simulink model "ADCS_r2017b_may6"  (R2018a)
settings: Solver=VariableStepAuto  StartTime=0.0  StopTime=10.0  RelTol=1e-3
undefined symbols (not defined in the file or in its folder): delta_t, SC, SS
libraries: sharedutil x3, vrlib x2
(part 1 of 2)
settings Model: Creator=azufall  LastModifiedBy=Hridu

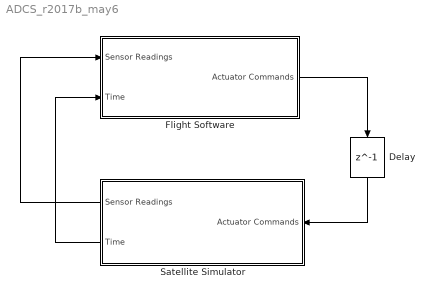
== system ADCS_r2017b_may6 ==
  Delay : Delay  DelayLength=1  InitialCondition=0
  Flight Software : Subsystem
  Satellite Simulator : Subsystem
  wires:
  Flight Software/1(Actuator Commands) -> Delay/1
  Satellite Simulator/2(Time) -> Flight Software/2(Time)
  Satellite Simulator/1(Sensor Readings) -> Flight Software/1(Sensor Readings)
  Delay/1 -> Satellite Simulator/1(Actuator Commands)

== system ADCS_r2017b_may6/Flight Software ==
  Sensor Readings : Inport
  Time : Inport  Port=2
  Bus Selector : BusSelector  OutputSignals=gyro meas,sun meas,star meas
  Resolution Error : Rounding
  Subsystems : Subsystem
  Thrust command : Gain
  Actuator Commands : Outport
  wires:
  Subsystems/1(RCS Command) -> Thrust command/1
  Sensor Readings/1 -> Bus Selector/1
  Bus Selector/1 -> Subsystems/1(Gyro)  "<gyro meas>"
  Bus Selector/3 -> Subsystems/3(Star Tracker)  "<star meas>"
  Time/1 -> Subsystems/4(Time)
  Thrust command/1 -> Resolution Error/1
  Resolution Error/1 -> Actuator Commands/1
  Bus Selector/2 -> Subsystems/2(Sun Sensor)  "<sun meas>"

== system ADCS_r2017b_may6/Satellite Simulator ==
  Actuator Commands : Inport
  Actuators : Subsystem
  Constant : Constant  Value=0
  Environment : Subsystem
  External Forces and Torques : Subsystem
  Kinematics : Subsystem
  Sensors : Subsystem
  Sum : Sum  Inputs=++|
  Sum1 : Sum  Inputs=++|
  Time Model : Subsystem
  Sensor Readings : Outport
  Time : Outport  Port=2
  wires:
  Kinematics/3(Omega) -> Sensors/3(w_body2eci)
  Sensors/1(Sensor Readings) -> Sensor Readings/1
  Time Model/1(JD) -> Kinematics/3(JD), Environment/1(Time), Time/1
  Environment/1(sun_eci) -> Sensors/2(Sun info), External Forces and Torques/4(sun_eci)
  Environment/2(moon_eci) -> External Forces and Torques/5(moon_eci)
  Environment/3(Mag) -> External Forces and Torques/6(Mag)
  External Forces and Torques/1(Ex Forces) -> Sum/2
  Sum/1 -> Kinematics/1(a_eci)
  External Forces and Torques/2(Ex Torques) -> Sum1/2
  Kinematics/2(Velocity) -> External Forces and Torques/2(Velocity)
  Kinematics/4(Coordinate Transforms) -> Environment/3(Coordinate Transforms), Sensors/4(Coordinate Transforms), Actuators/3(Coordinate Transforms), External Forces and Torques/3(Coordinate Transforms)
  Actuators/1(a_eci) -> Sum/1
  Actuators/2(torque_body) -> Sum1/1
  Sum1/1 -> Kinematics/2(Torque_body)
  Kinematics/1(Position) -> Sensors/1(Position), Environment/2(r_eci), External Forces and Torques/1(Position)
  Environment/4(Eclipse) -> Sensors/5(eclipse), External Forces and Torques/7(Eclipse)
  Kinematics/5(q) -> Sensors/6(q_eci2body)
  Actuator Commands/1 -> Actuators/1(RCS Command)
  Constant/1 -> Actuators/2(Other Actuator?)

== system ADCS_r2017b_may6/Flight Software/Subsystems ==
  Gyro : Inport
  Sun Sensor : Inport  Port=2
  Star Tracker : Inport  Port=3
  Time : Inport  Port=4
  Mode Selection : Subsystem
  RCS Controller : Subsystem
  Sensor Processing : Subsystem
  RCS Command : Outport
  wires:
  Gyro/1 -> Sensor Processing/1(Gyro_raw)
  Sun Sensor/1 -> Sensor Processing/2(Sun_raw)
  Star Tracker/1 -> Sensor Processing/3(Star_raw)
  Sensor Processing/1(Gyro_filtered) -> RCS Controller/2(Gyro), Mode Selection/1(Gyro)
  Sensor Processing/4(Eclipse) -> Mode Selection/2(Eclipse)
  Time/1 -> RCS Controller/6(Time), Mode Selection/3(Time)
  RCS Controller/1(RCS_Command) -> RCS Command/1
  Mode Selection/2(S/C Mode) -> RCS Controller/1(Mode)
  Mode Selection/1(Controller Gains) -> RCS Controller/5(Gains)
  Sensor Processing/3(Star_filtered) -> RCS Controller/4(Star)
  Sensor Processing/2(Sun_filtered) -> RCS Controller/3(Sun)

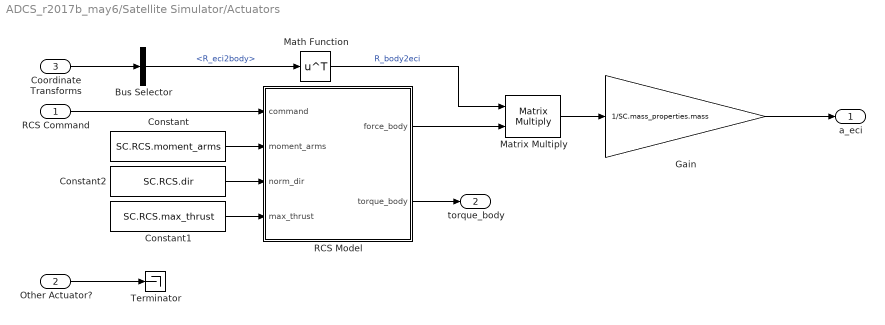
== system ADCS_r2017b_may6/Satellite Simulator/Actuators ==
  RCS Command : Inport
  Other Actuator? : Inport  Port=2
  Coordinate Transforms : Inport  Port=3
  Bus Selector : BusSelector  OutputSignals=R_eci2body
  Constant : Constant  Value=SC.RCS.moment_arms
  Constant1 : Constant  Value=SC.RCS.max_thrust
  Constant2 : Constant  Value=SC.RCS.dir
  Gain : Gain  Gain=1/SC.mass_properties.mass
  Math Function : Math  Operator=transpose  SaturateOnIntegerOverflow=on
  Matrix Multiply : Product  Multiplication=Matrix(*)
  RCS Model : MATLAB Function  TreatAsAtomicUnit=on
  Terminator : Terminator
  a_eci : Outport
  torque_body : Outport  Port=2
  wires:
  RCS Command/1 -> RCS Model/1(command)
  RCS Model/2(torque_body) -> torque_body/1
  Other Actuator?/1 -> Terminator/1
  Coordinate Transforms/1 -> Bus Selector/1
  Bus Selector/1 -> Math Function/1  "<R_eci2body>"
  RCS Model/1(force_body) -> Matrix Multiply/2
  Matrix Multiply/1 -> Gain/1
  Math Function/1 -> Matrix Multiply/1  "R_body2eci"
  Constant/1 -> RCS Model/2(moment_arms)
  Constant1/1 -> RCS Model/4(max_thrust)
  Constant2/1 -> RCS Model/3(norm_dir)
  Gain/1 -> a_eci/1

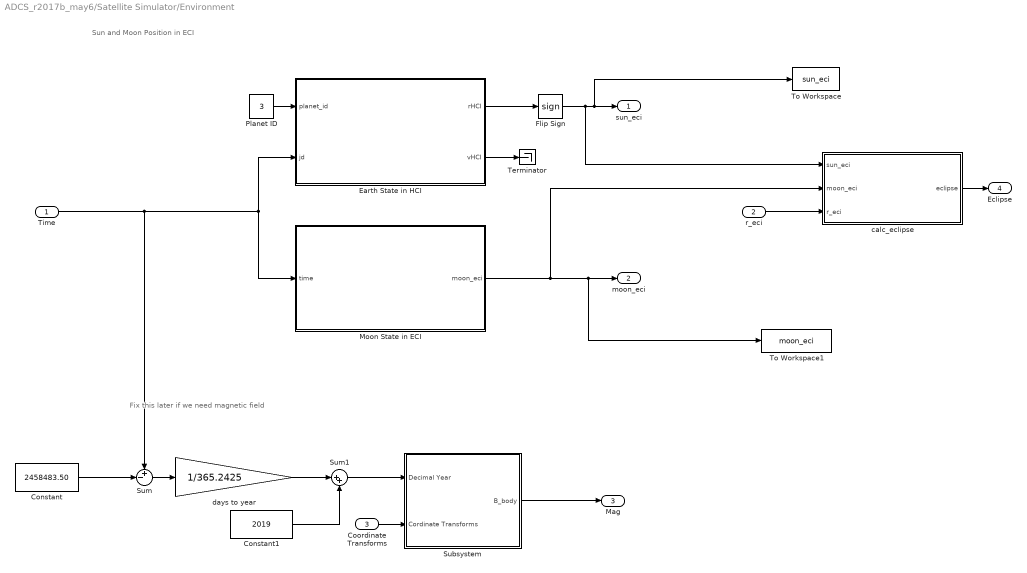
== system ADCS_r2017b_may6/Satellite Simulator/Environment ==
  note: Sun and Moon Position in ECI
  note: Fix this later if we need magnetic field
  Time : Inport
  r_eci : Inport  Port=2
  Coordinate Transforms : Inport  Port=3
  Constant : Constant  Value=2458483.50
  Constant1 : Constant  Value=2019
  Earth State in HCI : MATLAB Function  TreatAsAtomicUnit=on
  Flip Sign : Signum
  Moon State in ECI : MATLAB Function  TreatAsAtomicUnit=on
  Planet ID : Constant  Value=3
  Subsystem : Subsystem
  Sum : Sum  Inputs=+-|
  Sum1 : Sum  Inputs=|++
  Terminator : Terminator
  To Workspace : ToWorkspace  VariableName=sun_eci  SampleTime=-1
  To Workspace1 : ToWorkspace  VariableName=moon_eci  SampleTime=-1
  calc_eclipse : MATLAB Function  TreatAsAtomicUnit=on
  days to year : Gain  Gain=1/365.2425
  sun_eci : Outport
  moon_eci : Outport  Port=2
  Mag : Outport  Port=3
  Eclipse : Outport  Port=4
  wires:
  Moon State in ECI/1(moon_eci) -> calc_eclipse/2(moon_eci), To Workspace1/1, moon_eci/1
  Subsystem/1(B_body) -> Mag/1
  calc_eclipse/1(eclipse) -> Eclipse/1
  Time/1 -> Sum/1, Earth State in HCI/2(jd), Moon State in ECI/1(time)
  Planet ID/1 -> Earth State in HCI/1(planet_id)
  Earth State in HCI/1(rHCI) -> Flip Sign/1
  Flip Sign/1 -> calc_eclipse/1(sun_eci), To Workspace/1, sun_eci/1
  r_eci/1 -> calc_eclipse/3(r_eci)
  Earth State in HCI/2(vHCI) -> Terminator/1
  Sum/1 -> days to year/1
  Constant/1 -> Sum/2
  days to year/1 -> Sum1/1
  Sum1/1 -> Subsystem/1(Decimal Year)
  Constant1/1 -> Sum1/2
  Coordinate Transforms/1 -> Subsystem/2(Cordinate Transforms)

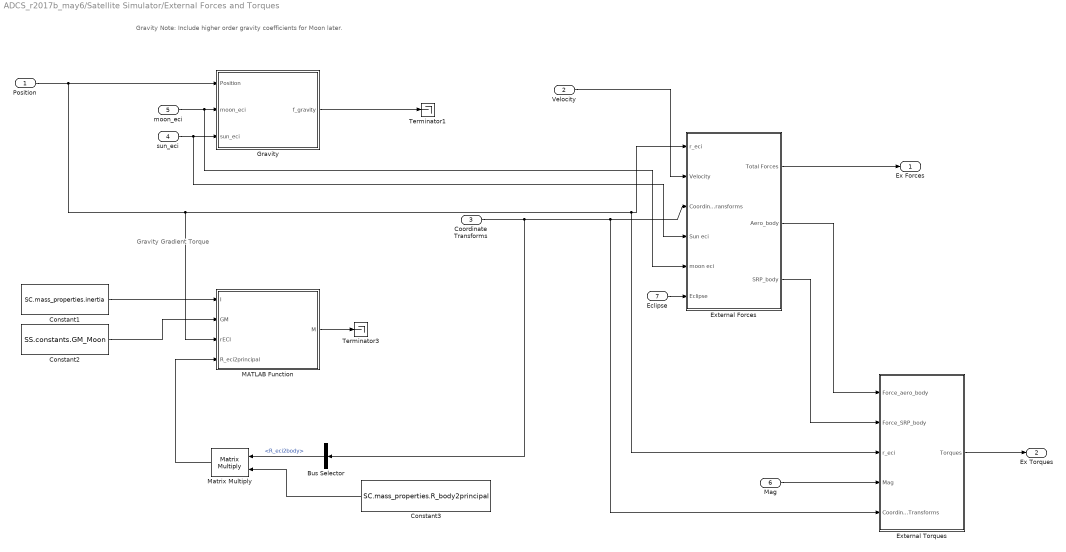
== system ADCS_r2017b_may6/Satellite Simulator/External Forces and Torques ==
  note: Gravity Gradient Torque
  note: Gravity
      |
      | Note: Include higher order gravity coefficients for Moon later.
  Position : Inport
  Velocity : Inport  Port=2
  Coordinate Transforms : Inport  Port=3
  sun_eci : Inport  Port=4
  moon_eci : Inport  Port=5
  Mag : Inport  Port=6
  Eclipse : Inport  Port=7
  Bus Selector : BusSelector  OutputSignals=R_eci2body
  Constant1 : Constant  Value=SC.mass_properties.inertia
  Constant2 : Constant  Value=SS.constants.GM_Moon
  Constant3 : Constant  Value=SC.mass_properties.R_body2principal
  External Forces : Subsystem
  External Torques : Subsystem
  Gravity : Subsystem
  MATLAB Function : MATLAB Function  TreatAsAtomicUnit=on
  Matrix Multiply : Product  Multiplication=Matrix(*)
  Terminator1 : Terminator
  Terminator3 : Terminator
  Ex Forces : Outport
  Ex Torques : Outport  Port=2
  wires:
  External Forces/2(Aero_body) -> External Torques/1(Force_aero_body)
  External Forces/3(SRP_body) -> External Torques/2(Force_SRP_body)
  Position/1 -> MATLAB Function/3(rECI), External Torques/3(r_eci), External Forces/1(r_eci), Gravity/1(Position)
  moon_eci/1 -> External Forces/5(moon eci), Gravity/2(moon_eci)
  sun_eci/1 -> External Forces/4(Sun eci), Gravity/3(sun_eci)
  Velocity/1 -> External Forces/2(Velocity)
  Coordinate Transforms/1 -> Bus Selector/1, External Torques/5(Coordinate Transforms), External Forces/3(Coordinate Transforms)
  MATLAB Function/1(M) -> Terminator3/1
  Constant1/1 -> MATLAB Function/1(I)
  Constant2/1 -> MATLAB Function/2(GM)
  Eclipse/1 -> External Forces/6(Eclipse)
  Mag/1 -> External Torques/4(Mag)
  Gravity/1(f_gravity) -> Terminator1/1
  External Forces/1(Total Forces) -> Ex Forces/1
  External Torques/1(Torques) -> Ex Torques/1
  Bus Selector/1 -> Matrix Multiply/1  "<R_eci2body>"
  Constant3/1 -> Matrix Multiply/2
  Matrix Multiply/1 -> MATLAB Function/4(R_eci2principal)

== system ADCS_r2017b_may6/Satellite Simulator/Kinematics ==
  a_eci : Inport
  Torque_body : Inport  Port=2
  JD : Inport  Port=3
  Calc Coordinate Transforms : Subsystem
  Position Kinematics : Subsystem
  Rotation Kinematics : Subsystem
  TEST POSITION KINEMATICS : Subsystem  Commented=on
  Position : Outport
  Velocity : Outport  Port=2
  Omega : Outport  Port=3
  Coordinate Transforms : Outport  Port=4
  q : Outport  Port=5
  wires:
  a_eci/1 -> Position Kinematics/1(a_eci)
  Torque_body/1 -> Rotation Kinematics/1(torque_body)
  Rotation Kinematics/2(w_body_eci) -> Omega/1
  Rotation Kinematics/1(q) -> q/1, Calc Coordinate Transforms/4(Attitude)
  Position Kinematics/1(r_eci) -> Position/1, Calc Coordinate Transforms/1(r_eci)
  Position Kinematics/2(v_eci) -> Velocity/1, Calc Coordinate Transforms/2(Velocity)
  Calc Coordinate Transforms/1(Coordinate Transforms) -> Coordinate Transforms/1
  JD/1 -> Calc Coordinate Transforms/3(JD)

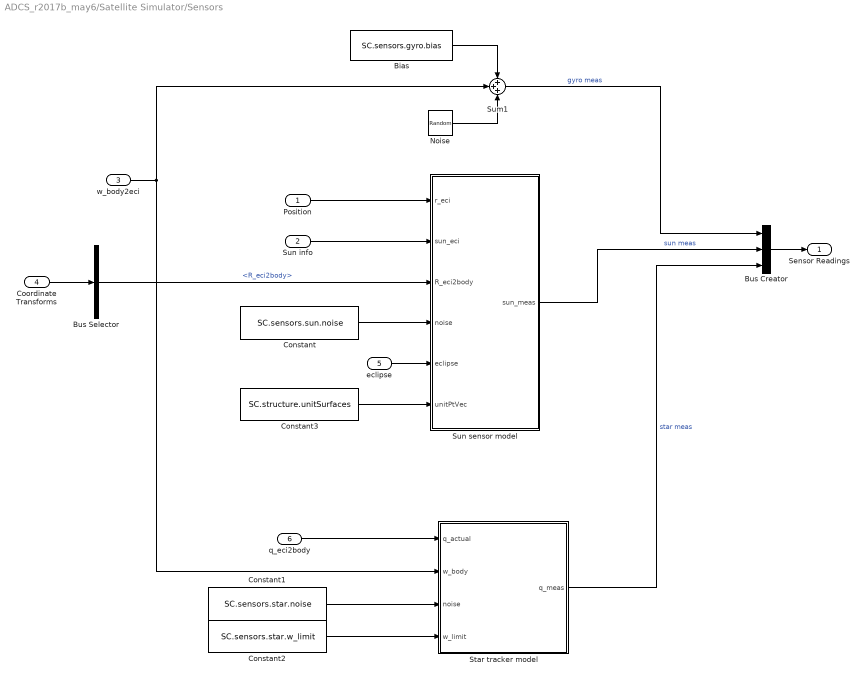
== system ADCS_r2017b_may6/Satellite Simulator/Sensors ==
  Position : Inport
  Sun info : Inport  Port=2
  w_body2eci : Inport  Port=3
  Coordinate Transforms : Inport  Port=4
  eclipse : Inport  Port=5
  q_eci2body : Inport  Port=6
  Bias : Constant  Value=SC.sensors.gyro.bias
  Bus Creator : BusCreator  Inputs=3
  Bus Selector : BusSelector  OutputSignals=R_eci2body
  Constant : Constant  Value=SC.sensors.sun.noise
  Constant1 : Constant  Value=SC.sensors.star.noise
  Constant2 : Constant  Value=SC.sensors.star.w_limit
  Constant3 : Constant  Value=SC.structure.unitSurfaces
  Noise : RandomNumber  Variance=SC.sensors.gyro.noise  SampleTime=0.1
  Star tracker model : MATLAB Function  TreatAsAtomicUnit=on
  Sum1 : Sum  Inputs=+++
  Sun sensor model : MATLAB Function  TreatAsAtomicUnit=on
  Sensor Readings : Outport
  wires:
  Bus Creator/1 -> Sensor Readings/1
  Star tracker model/1(q_meas) -> Bus Creator/3  "star meas"
  Sun info/1 -> Sun sensor model/2(sun_eci)
  Position/1 -> Sun sensor model/1(r_eci)
  Constant/1 -> Sun sensor model/4(noise)
  Sun sensor model/1(sun_meas) -> Bus Creator/2  "sun meas"
  Noise/1 -> Sum1/3
  Bias/1 -> Sum1/1
  w_body2eci/1 -> Star tracker model/2(w_body), Sum1/2
  Sum1/1 -> Bus Creator/1  "gyro meas"
  Constant1/1 -> Star tracker model/3(noise)
  Constant2/1 -> Star tracker model/4(w_limit)
  eclipse/1 -> Sun sensor model/5(eclipse)
  Coordinate Transforms/1 -> Bus Selector/1
  Bus Selector/1 -> Sun sensor model/3(R_eci2body)  "<R_eci2body>"
  Constant3/1 -> Sun sensor model/6(unitPtVec)
  q_eci2body/1 -> Star tracker model/1(q_actual)

== system ADCS_r2017b_may6/Satellite Simulator/Time Model ==
  Constant : Constant  Value=SC.initial_state.date  VectorParams1D=off
  Constant1 : Constant  Value=delta_t
  Date2JD : MATLAB Function  TreatAsAtomicUnit=on
  Delay : Delay  DelayLength=1  InitialConditionSource=Input port  InitialCondition=0
      settings: InputPortMap=u0,p4
  Sum : Sum  Inputs=|++
  To Workspace : ToWorkspace  VariableName=JD  SampleTime=-1
  days per second : Gain  Gain=1/(24*60*60)
  JD : Outport
  wires:
  Sum/1 -> To Workspace/1, JD/1, Delay/1
  Constant1/1 -> days per second/1
  Delay/1 -> Sum/1
  Constant/1 -> Date2JD/1(date)
  Date2JD/1(JD) -> Delay/2
  days per second/1 -> Sum/2

== system ADCS_r2017b_may6/Flight Software/Subsystems/Mode Selection ==
  Gyro : Inport
  Eclipse : Inport  Port=2
  Time : Inport  Port=3
  3_axis_gains : Constant  Value=SC.ax3.gains
  3_axis_gains1 : Constant  Value=SC.spin.gains
  3_axis_gains2 : Constant  Value=SC.ax3.time_constant
  3_axis_gains3 : Constant  Value=SC.spin.time_constant
  3_axis_gains4 : Constant  Value=SC.spin_up.time_constant
  3_axis_gains5 : Constant  Value=SC.spin_up.gains
  MATLAB Function : MATLAB Function  TreatAsAtomicUnit=on
  Controller Gains : Outport
  S/C Mode : Outport  Port=2
  wires:
  Time/1 -> MATLAB Function/3(JD)
  Gyro/1 -> MATLAB Function/1(gyro)
  Eclipse/1 -> MATLAB Function/2(eclipse)
  MATLAB Function/1(gains) -> Controller Gains/1
  MATLAB Function/2(mode) -> S/C Mode/1
  3_axis_gains/1 -> MATLAB Function/4(a)
  3_axis_gains2/1 -> MATLAB Function/5(b)
  3_axis_gains1/1 -> MATLAB Function/6(c)
  3_axis_gains3/1 -> MATLAB Function/7(d)
  3_axis_gains5/1 -> MATLAB Function/8(e)
  3_axis_gains4/1 -> MATLAB Function/9(f)

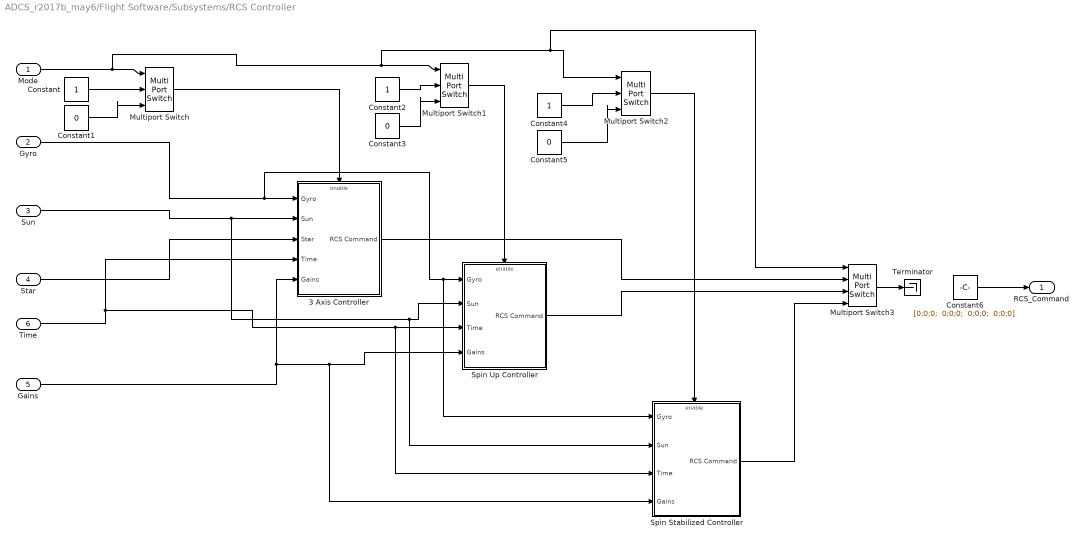
== system ADCS_r2017b_may6/Flight Software/Subsystems/RCS Controller ==
  Mode : Inport
  Gyro : Inport  Port=2
  Sun : Inport  Port=3
  Star : Inport  Port=4
  Gains : Inport  Port=5
  Time : Inport  Port=6
  3 Axis Controller : Subsystem  TreatAsAtomicUnit=on
  Constant : Constant
  Constant1 : Constant  Value=0
  Constant2 : Constant
  Constant3 : Constant  Value=0
  Constant4 : Constant
  Constant5 : Constant  Value=0
  Constant6 : Constant  Value="[0;0;0;  0;0;0;  0;0;0;  0;0;0]"
  Multiport Switch : MultiPortSwitch  Inputs=2
  Multiport Switch1 : MultiPortSwitch  Inputs=2
  Multiport Switch2 : MultiPortSwitch  Inputs=2
  Multiport Switch3 : MultiPortSwitch
  Spin Stabilized Controller : Subsystem  TreatAsAtomicUnit=on
  Spin Up Controller : Subsystem  TreatAsAtomicUnit=on
  Terminator : Terminator
  RCS_Command : Outport
  wires:
  Multiport Switch/1 -> 3 Axis Controller/Enable
  Multiport Switch1/1 -> Spin Up Controller/Enable
  Multiport Switch2/1 -> Spin Stabilized Controller/Enable
  Mode/1 -> Multiport Switch3/1, Multiport Switch2/1, Multiport Switch1/1, Multiport Switch/1
  Gyro/1 -> Spin Stabilized Controller/1(Gyro), Spin Up Controller/1(Gyro), 3 Axis Controller/1(Gyro)
  Sun/1 -> Spin Stabilized Controller/2(Sun), Spin Up Controller/2(Sun), 3 Axis Controller/2(Sun)
  Star/1 -> 3 Axis Controller/3(Star)
  Time/1 -> Spin Stabilized Controller/3(Time), Spin Up Controller/3(Time), 3 Axis Controller/4(Time)
  Gains/1 -> Spin Stabilized Controller/4(Gains), Spin Up Controller/4(Gains), 3 Axis Controller/5(Gains)
  3 Axis Controller/1(RCS Command) -> Multiport Switch3/2
  Spin Up Controller/1(RCS Command) -> Multiport Switch3/3
  Spin Stabilized Controller/1(RCS Command) -> Multiport Switch3/4
  Constant/1 -> Multiport Switch/2
  Constant1/1 -> Multiport Switch/3
  Constant2/1 -> Multiport Switch1/2
  Constant3/1 -> Multiport Switch1/3
  Constant4/1 -> Multiport Switch2/2
  Constant5/1 -> Multiport Switch2/3
  Multiport Switch3/1 -> Terminator/1
  Constant6/1 -> RCS_Command/1

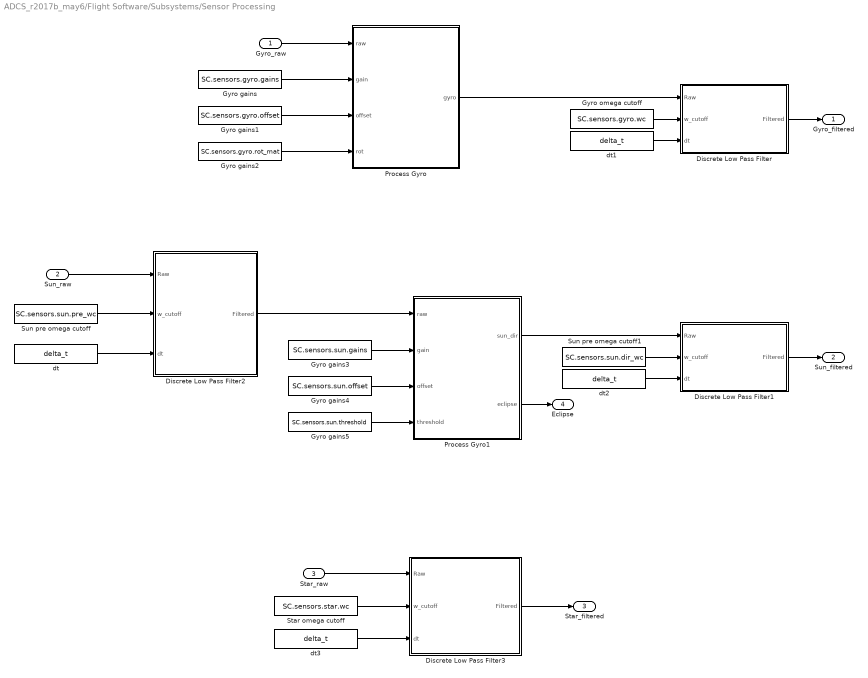
== system ADCS_r2017b_may6/Flight Software/Subsystems/Sensor Processing ==
  Gyro_raw : Inport
  Sun_raw : Inport  Port=2
  Star_raw : Inport  Port=3
  Discrete Low Pass Filter : Subsystem
  Discrete Low Pass Filter1 : Subsystem
  Discrete Low Pass Filter2 : Subsystem
  Discrete Low Pass Filter3 : Subsystem
  Gyro gains : Constant  Value=SC.sensors.gyro.gains
  Gyro gains1 : Constant  Value=SC.sensors.gyro.offset
  Gyro gains2 : Constant  Value=SC.sensors.gyro.rot_mat
  Gyro gains3 : Constant  Value=SC.sensors.sun.gains
  Gyro gains4 : Constant  Value=SC.sensors.sun.offset
  Gyro gains5 : Constant  Value=SC.sensors.sun.threshold
  Gyro omega cutoff : Constant  Value=SC.sensors.gyro.wc
  Process Gyro : MATLAB Function  TreatAsAtomicUnit=on
  Process Gyro1 : MATLAB Function  TreatAsAtomicUnit=on
  Star omega cutoff : Constant  Value=SC.sensors.star.wc
  Sun pre omega cutoff : Constant  Value=SC.sensors.sun.pre_wc
  Sun pre omega cutoff1 : Constant  Value=SC.sensors.sun.dir_wc
  dt{,1..3} (4 alike) : Constant  Value=delta_t
  Gyro_filtered : Outport
  Sun_filtered : Outport  Port=2
  Star_filtered : Outport  Port=3
  Eclipse : Outport  Port=4
  wires:
  Gyro_raw/1 -> Process Gyro/1(raw)
  Gyro gains/1 -> Process Gyro/2(gain)
  Gyro gains1/1 -> Process Gyro/3(offset)
  Gyro gains2/1 -> Process Gyro/4(rot)
  Discrete Low Pass Filter/1(Filtered) -> Gyro_filtered/1
  Process Gyro/1(gyro) -> Discrete Low Pass Filter/1(Raw)
  Gyro omega cutoff/1 -> Discrete Low Pass Filter/2(w_cutoff)
  dt1/1 -> Discrete Low Pass Filter/3(dt)
  Sun_raw/1 -> Discrete Low Pass Filter2/1(Raw)
  Discrete Low Pass Filter2/1(Filtered) -> Process Gyro1/1(raw)
  Discrete Low Pass Filter1/1(Filtered) -> Sun_filtered/1
  Process Gyro1/1(sun_dir) -> Discrete Low Pass Filter1/1(Raw)
  Process Gyro1/2(eclipse) -> Eclipse/1
  Sun pre omega cutoff/1 -> Discrete Low Pass Filter2/2(w_cutoff)
  dt/1 -> Discrete Low Pass Filter2/3(dt)
  Gyro gains3/1 -> Process Gyro1/2(gain)
  Gyro gains4/1 -> Process Gyro1/3(offset)
  Gyro gains5/1 -> Process Gyro1/4(threshold)
  Sun pre omega cutoff1/1 -> Discrete Low Pass Filter1/2(w_cutoff)
  dt2/1 -> Discrete Low Pass Filter1/3(dt)
  Star_raw/1 -> Discrete Low Pass Filter3/1(Raw)
  Discrete Low Pass Filter3/1(Filtered) -> Star_filtered/1
  Star omega cutoff/1 -> Discrete Low Pass Filter3/2(w_cutoff)
  dt3/1 -> Discrete Low Pass Filter3/3(dt)

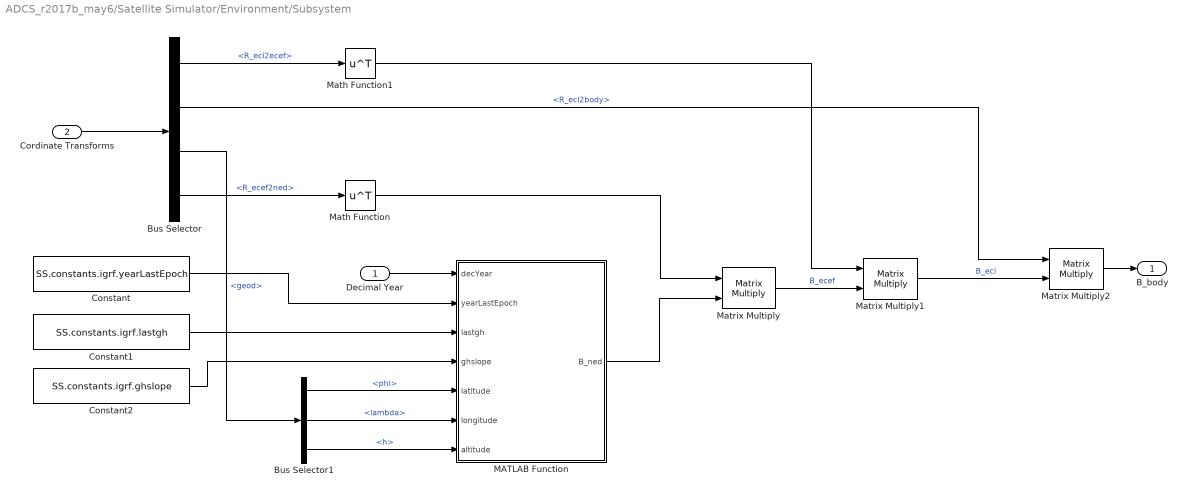
== system ADCS_r2017b_may6/Satellite Simulator/Environment/Subsystem ==
  Decimal Year : Inport
  Cordinate Transforms : Inport  Port=2
  Bus Selector : BusSelector  OutputSignals=R_eci2ecef,R_eci2body,geod,R_ecef2ned
  Bus Selector1 : BusSelector  OutputSignals=phi,lambda,h
  Constant : Constant  Value=SS.constants.igrf.yearLastEpoch
  Constant1 : Constant  Value=SS.constants.igrf.lastgh
  Constant2 : Constant  Value=SS.constants.igrf.ghslope
  MATLAB Function : MATLAB Function  TreatAsAtomicUnit=on
  Math Function : Math  Operator=transpose  SaturateOnIntegerOverflow=on
  Math Function1 : Math  Operator=transpose  SaturateOnIntegerOverflow=on
  Matrix Multiply : Product  Multiplication=Matrix(*)
  Matrix Multiply1 : Product  Multiplication=Matrix(*)
  Matrix Multiply2 : Product  Multiplication=Matrix(*)
  B_body : Outport
  wires:
  Cordinate Transforms/1 -> Bus Selector/1
  Bus Selector/4 -> Math Function/1  "<R_ecef2ned>"
  MATLAB Function/1(B_ned) -> Matrix Multiply/2
  Math Function/1 -> Matrix Multiply/1
  Bus Selector/3 -> Bus Selector1/1  "<geod>"
  Bus Selector/2 -> Matrix Multiply2/1  "<R_eci2body>"
  Bus Selector/1 -> Math Function1/1  "<R_eci2ecef>"
  Matrix Multiply/1 -> Matrix Multiply1/2  "B_ecef"
  Matrix Multiply1/1 -> Matrix Multiply2/2  "B_eci"
  Matrix Multiply2/1 -> B_body/1
  Math Function1/1 -> Matrix Multiply1/1
  Decimal Year/1 -> MATLAB Function/1(decYear)
  Bus Selector1/3 -> MATLAB Function/7(altitude)  "<h>"
  Bus Selector1/1 -> MATLAB Function/5(latitude)  "<phi>"
  Bus Selector1/2 -> MATLAB Function/6(longitude)  "<lambda>"
  Constant/1 -> MATLAB Function/2(yearLastEpoch)
  Constant1/1 -> MATLAB Function/3(lastgh)
  Constant2/1 -> MATLAB Function/4(ghslope)

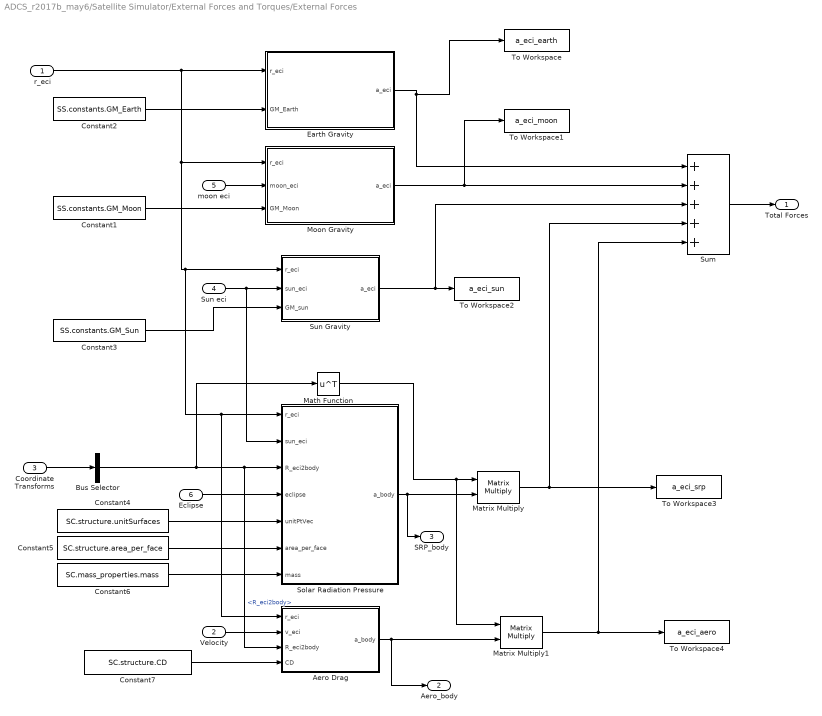
== system ADCS_r2017b_may6/Satellite Simulator/External Forces and Torques/External Forces ==
  r_eci : Inport
  Velocity : Inport  Port=2
  Coordinate Transforms : Inport  Port=3
  Sun eci : Inport  Port=4
  moon eci : Inport  Port=5
  Eclipse : Inport  Port=6
  Aero Drag : MATLAB Function  TreatAsAtomicUnit=on
  Bus Selector : BusSelector  OutputSignals=R_eci2body
  Constant1 : Constant  Value=SS.constants.GM_Moon
  Constant2 : Constant  Value=SS.constants.GM_Earth
  Constant3 : Constant  Value=SS.constants.GM_Sun
  Constant4 : Constant  Value=SC.structure.unitSurfaces
  Constant5 : Constant  Value=SC.structure.area_per_face
  Constant6 : Constant  Value=SC.mass_properties.mass
  Constant7 : Constant  Value=SC.structure.CD
  Earth Gravity : MATLAB Function  TreatAsAtomicUnit=on
  Math Function : Math  Operator=transpose  SaturateOnIntegerOverflow=on
  Matrix Multiply : Product  Multiplication=Matrix(*)
  Matrix Multiply1 : Product  Multiplication=Matrix(*)
  Moon Gravity : MATLAB Function  TreatAsAtomicUnit=on
  Solar Radiation Pressure : MATLAB Function  TreatAsAtomicUnit=on
  Sum : Sum  Inputs=+++++
  Sun Gravity : MATLAB Function  TreatAsAtomicUnit=on
  To Workspace : ToWorkspace  VariableName=a_eci_earth  SampleTime=-1
  To Workspace1 : ToWorkspace  VariableName=a_eci_moon  SampleTime=-1
  To Workspace2 : ToWorkspace  VariableName=a_eci_sun  SampleTime=-1
  To Workspace3 : ToWorkspace  VariableName=a_eci_srp  SampleTime=-1
  To Workspace4 : ToWorkspace  VariableName=a_eci_aero  SampleTime=-1
  Total Forces : Outport
  Aero_body : Outport  Port=2
  SRP_body : Outport  Port=3
  wires:
  Sun eci/1 -> Solar Radiation Pressure/2(sun_eci), Sun Gravity/2(sun_eci)
  Solar Radiation Pressure/1(a_body) -> SRP_body/1, Matrix Multiply/2
  Sum/1 -> Total Forces/1
  Earth Gravity/1(a_eci) -> To Workspace/1, Sum/1
  Sun Gravity/1(a_eci) -> To Workspace2/1, Sum/3
  Velocity/1 -> Aero Drag/2(v_eci)
  Coordinate Transforms/1 -> Bus Selector/1
  Moon Gravity/1(a_eci) -> To Workspace1/1, Sum/2
  r_eci/1 -> Aero Drag/1(r_eci), Solar Radiation Pressure/1(r_eci), Sun Gravity/1(r_eci), Moon Gravity/1(r_eci), Earth Gravity/1(r_eci)
  Bus Selector/1 -> Math Function/1, Aero Drag/3(R_eci2body), Solar Radiation Pressure/3(R_eci2body)  "<R_eci2body>"
  moon eci/1 -> Moon Gravity/2(moon_eci)
  Constant1/1 -> Moon Gravity/3(GM_Moon)
  Constant2/1 -> Earth Gravity/2(GM_Earth)
  Constant3/1 -> Sun Gravity/3(GM_sun)
  Eclipse/1 -> Solar Radiation Pressure/4(eclipse)
  Constant4/1 -> Solar Radiation Pressure/5(unitPtVec)
  Constant5/1 -> Solar Radiation Pressure/6(area_per_face)
  Constant6/1 -> Solar Radiation Pressure/7(mass)
  Constant7/1 -> Aero Drag/4(CD)
  Matrix Multiply/1 -> To Workspace3/1, Sum/4
  Math Function/1 -> Matrix Multiply1/1, Matrix Multiply/1
  Aero Drag/1(a_body) -> Aero_body/1, Matrix Multiply1/2
  Matrix Multiply1/1 -> To Workspace4/1, Sum/5

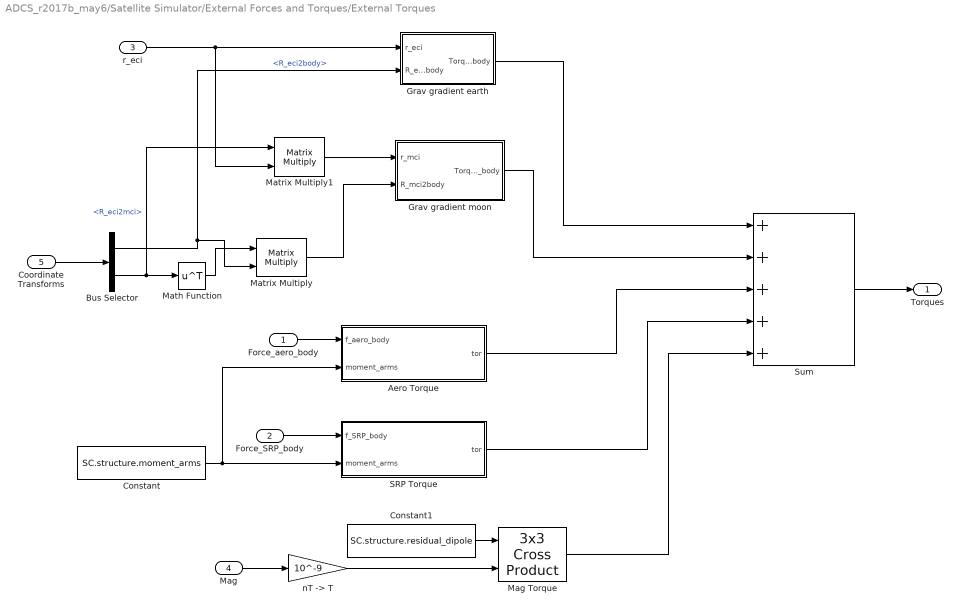
== system ADCS_r2017b_may6/Satellite Simulator/External Forces and Torques/External Torques ==
  Force_aero_body : Inport
  Force_SRP_body : Inport  Port=2
  r_eci : Inport  Port=3
  Mag : Inport  Port=4
  Coordinate Transforms : Inport  Port=5
  Aero Torque : MATLAB Function  TreatAsAtomicUnit=on
  Bus Selector : BusSelector  OutputSignals=R_eci2body,R_eci2mci
  Constant : Constant  Value=SC.structure.moment_arms
  Constant1 : Constant  Value=SC.structure.residual_dipole
  Grav gradient earth : Subsystem
  Grav gradient moon : Subsystem
  Mag Torque : sharedutil/3x3 Cross Product  aMode=aMode
      settings: SourceProductBaseCode=AE
  Math Function : Math  Operator=transpose  SaturateOnIntegerOverflow=on
  Matrix Multiply : Product  Multiplication=Matrix(*)
  Matrix Multiply1 : Product  Multiplication=Matrix(*)
  SRP Torque : MATLAB Function  TreatAsAtomicUnit=on
  Sum : Sum  Inputs=5
  "nT -> T" : Gain  Gain=10^-9
  Torques : Outport
  wires:
  r_eci/1 -> Matrix Multiply1/2, Grav gradient earth/1(r_eci)
  Sum/1 -> Torques/1
  Grav gradient earth/1(Torque_body) -> Sum/1
  Grav gradient moon/1(Torque_body) -> Sum/2
  Aero Torque/1(tor) -> Sum/3
  Force_aero_body/1 -> Aero Torque/1(f_aero_body)
  Force_SRP_body/1 -> SRP Torque/1(f_SRP_body)
  SRP Torque/1(tor) -> Sum/4
  Mag Torque/1 -> Sum/5
  Mag/1 -> "nT -> T"/1
  Constant/1 -> Aero Torque/2(moment_arms), SRP Torque/2(moment_arms)
  Constant1/1 -> Mag Torque/1
  "nT -> T"/1 -> Mag Torque/2
  Coordinate Transforms/1 -> Bus Selector/1
  Bus Selector/1 -> Grav gradient earth/2(R_eci2body), Matrix Multiply/2  "<R_eci2body>"
  Bus Selector/2 -> Matrix Multiply1/1, Math Function/1  "<R_eci2mci>"
  Math Function/1 -> Matrix Multiply/1
  Matrix Multiply/1 -> Grav gradient moon/2(R_mci2body)
  Matrix Multiply1/1 -> Grav gradient moon/1(r_mci)

== system ADCS_r2017b_may6/Satellite Simulator/External Forces and Torques/Gravity ==
  note: Forces due to Point Mass Gravity
      |
      | Note: all computed in the inertial reference frames
  Position : Inport
  moon_eci : Inport  Port=2
  sun_eci : Inport  Port=3
  Constant : Constant  Value=SS.constants.GM_Earth
  Constant1 : Constant  Value=SS.constants.GM_Moon
  Constant2 : Constant  Value=SS.constants.GM_Sun
  Earth Gravity : MATLAB Function  TreatAsAtomicUnit=on
  Moon Gravity : MATLAB Function  TreatAsAtomicUnit=on
  Subtract : Sum  Inputs=+-
  Subtract1 : Sum  Inputs=+-
  Sum : Sum  Inputs=+++
  Sun Gravity : MATLAB Function  TreatAsAtomicUnit=on
  f_gravity : Outport
  wires:
  Position/1 -> Earth Gravity/1(r_eci), Subtract/1, Subtract1/1
  Sum/1 -> f_gravity/1
  Earth Gravity/1(f_Earth) -> Sum/1
  Sun Gravity/1(f_Sun) -> Sum/3
  Moon Gravity/1(f_Moon) -> Sum/2
  moon_eci/1 -> Subtract/2
  Subtract/1 -> Moon Gravity/1(r_mci)
  Subtract1/1 -> Sun Gravity/1(r_hci)
  sun_eci/1 -> Subtract1/2
  Constant/1 -> Earth Gravity/2(GM_Earth)
  Constant1/1 -> Moon Gravity/2(GM_Moon)
  Constant2/1 -> Sun Gravity/2(GM_Sun)

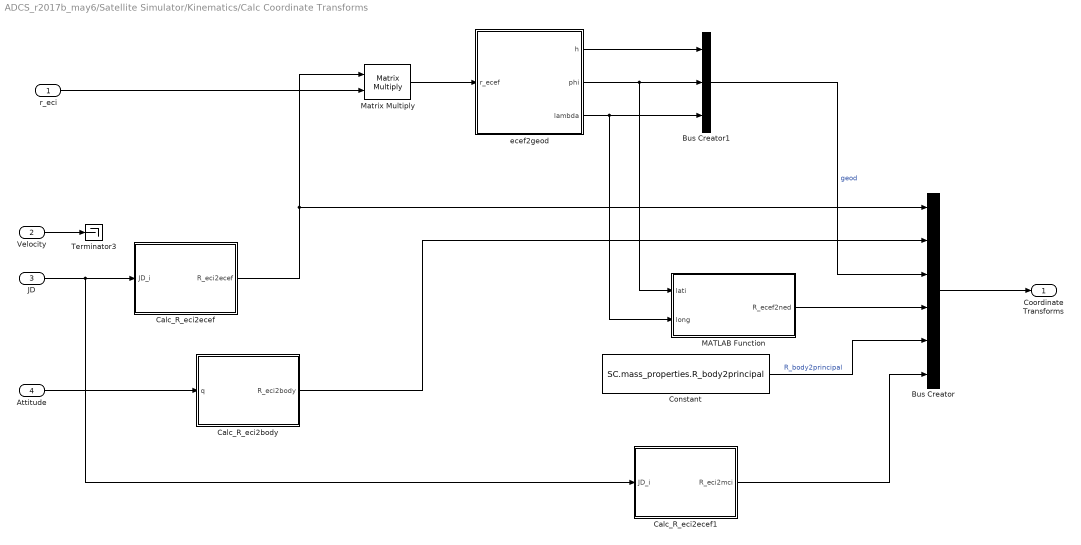
== system ADCS_r2017b_may6/Satellite Simulator/Kinematics/Calc Coordinate Transforms ==
  r_eci : Inport
  Velocity : Inport  Port=2
  JD : Inport  Port=3
  Attitude : Inport  Port=4
  Bus Creator : BusCreator  Inputs=6
  Bus Creator1 : BusCreator  Inputs=3
  Calc_R_eci2body : MATLAB Function  TreatAsAtomicUnit=on
  Calc_R_eci2ecef : MATLAB Function  TreatAsAtomicUnit=on
  Calc_R_eci2ecef1 : MATLAB Function  TreatAsAtomicUnit=on
  Constant : Constant  Value=SC.mass_properties.R_body2principal
  MATLAB Function : MATLAB Function  TreatAsAtomicUnit=on
  Matrix Multiply : Product  Multiplication=Matrix(*)
  Terminator3 : Terminator
  ecef2geod : MATLAB Function  TreatAsAtomicUnit=on
  Coordinate Transforms : Outport
  wires:
  Bus Creator/1 -> Coordinate Transforms/1
  Attitude/1 -> Calc_R_eci2body/1(q)
  JD/1 -> Calc_R_eci2ecef1/1(JD_i), Calc_R_eci2ecef/1(JD_i)
  r_eci/1 -> Matrix Multiply/2
  Matrix Multiply/1 -> ecef2geod/1(r_ecef)
  Calc_R_eci2ecef/1(R_eci2ecef) -> Matrix Multiply/1, Bus Creator/1
  ecef2geod/1(h) -> Bus Creator1/1
  ecef2geod/2(phi) -> MATLAB Function/1(lati), Bus Creator1/2
  ecef2geod/3(lambda) -> MATLAB Function/2(long), Bus Creator1/3
  Calc_R_eci2body/1(R_eci2body) -> Bus Creator/2
  Velocity/1 -> Terminator3/1
  Bus Creator1/1 -> Bus Creator/3  "geod"
  MATLAB Function/1(R_ecef2ned) -> Bus Creator/4
  Constant/1 -> Bus Creator/5  "R_body2principal"
  Calc_R_eci2ecef1/1(R_eci2mci) -> Bus Creator/6

== system ADCS_r2017b_may6/Satellite Simulator/Kinematics/Position Kinematics ==
  a_eci : Inport
  Adams Bashforth Integration : Subsystem
  Adams Bashforth Integration1 : Subsystem
  Constant : Constant  Value=SC.initial_state.r_eci
  Constant1 : Constant  Value=SC.initial_state.v_eci
  Constant2 : Constant  Value=delta_t
  To Workspace : ToWorkspace  VariableName=r_eci  SampleTime=-1
  To Workspace1 : ToWorkspace  VariableName=v_eci  SampleTime=-1
  r_eci : Outport
  v_eci : Outport  Port=2
  wires:
  a_eci/1 -> Adams Bashforth Integration1/2(x_dot)
  Constant2/1 -> Adams Bashforth Integration1/3(dt), Adams Bashforth Integration/3(dt)
  Constant/1 -> Adams Bashforth Integration/1(x_initial)
  Constant1/1 -> Adams Bashforth Integration1/1(x_initial)
  Adams Bashforth Integration1/1(x) -> To Workspace1/1, v_eci/1, Adams Bashforth Integration/2(x_dot)
  Adams Bashforth Integration/1(x) -> To Workspace/1, r_eci/1

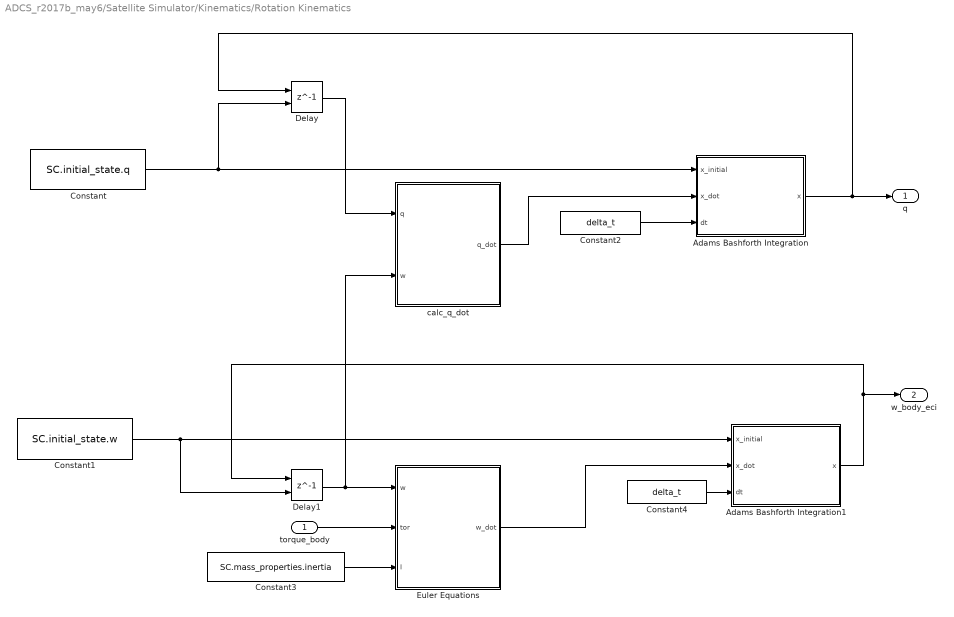
== system ADCS_r2017b_may6/Satellite Simulator/Kinematics/Rotation Kinematics ==
  torque_body : Inport
  Adams Bashforth Integration : Subsystem
  Adams Bashforth Integration1 : Subsystem
  Constant : Constant  Value=SC.initial_state.q
  Constant1 : Constant  Value=SC.initial_state.w
  Constant2 : Constant  Value=delta_t
  Constant3 : Constant  Value=SC.mass_properties.inertia
  Constant4 : Constant  Value=delta_t
  Delay : Delay  DelayLength=1  InitialConditionSource=Input port  InitialCondition=0
      settings: InputPortMap=u0,p4
  Delay1 : Delay  DelayLength=1  InitialConditionSource=Input port  InitialCondition=0
      settings: InputPortMap=u0,p4
  Euler Equations : MATLAB Function  TreatAsAtomicUnit=on
  calc_q_dot : MATLAB Function  TreatAsAtomicUnit=on
  q : Outport
  w_body_eci : Outport  Port=2
  wires:
  Constant/1 -> Delay/2, Adams Bashforth Integration/1(x_initial)
  Constant2/1 -> Adams Bashforth Integration/3(dt)
  Adams Bashforth Integration/1(x) -> q/1, Delay/1
  calc_q_dot/1(q_dot) -> Adams Bashforth Integration/2(x_dot)
  Delay/1 -> calc_q_dot/1(q)
  Constant1/1 -> Adams Bashforth Integration1/1(x_initial), Delay1/2
  Adams Bashforth Integration1/1(x) -> w_body_eci/1, Delay1/1
  torque_body/1 -> Euler Equations/2(tor)
  Euler Equations/1(w_dot) -> Adams Bashforth Integration1/2(x_dot)
  Constant3/1 -> Euler Equations/3(I)
  Delay1/1 -> calc_q_dot/2(w), Euler Equations/1(w)
  Constant4/1 -> Adams Bashforth Integration1/3(dt)

== system ADCS_r2017b_may6/Satellite Simulator/Kinematics/TEST POSITION KINEMATICS ==
  a_eci : Inport
  Constant3 : Constant  Value=SC.initial_state.r_eci
  Constant4 : Constant  Value=SC.initial_state.v_eci
  Integrator : Integrator  InitialConditionSource=external
  Integrator1 : Integrator  InitialConditionSource=external
  r_eci : Outport
  v_eci : Outport  Port=2
  wires:
  Constant4/1 -> Integrator/2
  a_eci/1 -> Integrator/1
  Integrator/1 -> v_eci/1, Integrator1/1
  Constant3/1 -> Integrator1/2
  Integrator1/1 -> r_eci/1

== system ADCS_r2017b_may6/Flight Software/Subsystems/RCS Controller/3 Axis Controller ==
  Gyro : Inport
  Sun : Inport  Port=2
  Star : Inport  Port=3
  Time : Inport  Port=4
  Gains : Inport  Port=5
  Enable : EnablePort
  RCS Command : Outport
  wires:
  Gyro/1 -> RCS Command/1

== system ADCS_r2017b_may6/Flight Software/Subsystems/RCS Controller/Spin Stabilized Controller ==
  Gyro : Inport
  Sun : Inport  Port=2
  Time : Inport  Port=3
  Gains : Inport  Port=4
  Enable : EnablePort
  RCS Command : Outport
  wires:
  Gyro/1 -> RCS Command/1

== system ADCS_r2017b_may6/Flight Software/Subsystems/RCS Controller/Spin Up Controller ==
  Gyro : Inport
  Sun : Inport  Port=2
  Time : Inport  Port=3
  Gains : Inport  Port=4
  Enable : EnablePort
  RCS Command : Outport
  wires:
  Gyro/1 -> RCS Command/1

== system ADCS_r2017b_may6/Flight Software/Subsystems/Sensor Processing/Discrete Low Pass Filter ==
  Raw : Inport
  w_cutoff : Inport  Port=2
  dt : Inport  Port=3
  Constant1 : Constant
  Delay : Delay  DelayLength=1  InitialCondition=0
  Divide : Product  Inputs=**
  Exp : Math  SaturateOnIntegerOverflow=on
  Gain : Gain  Gain=-1
  Product : Product
  Product1 : Product
  Sum : Sum  Inputs=|++
  Sum2 : Sum  Inputs=+-
  Filtered : Outport
  wires:
  w_cutoff/1 -> Divide/1
  dt/1 -> Divide/2
  Divide/1 -> Gain/1
  Raw/1 -> Product/1
  Product/1 -> Sum/1
  Sum/1 -> Delay/1, Filtered/1
  Product1/1 -> Sum/2
  Gain/1 -> Exp/1
  Exp/1 -> Product1/1, Sum2/2  "Alpha"
  Constant1/1 -> Sum2/1
  Sum2/1 -> Product/2
  Delay/1 -> Product1/2

== system ADCS_r2017b_may6/Flight Software/Subsystems/Sensor Processing/Discrete Low Pass Filter1 ==
  Raw : Inport
  w_cutoff : Inport  Port=2
  dt : Inport  Port=3
  Constant1 : Constant
  Delay : Delay  DelayLength=1  InitialCondition=0
  Divide : Product  Inputs=**
  Exp : Math  SaturateOnIntegerOverflow=on
  Gain : Gain  Gain=-1
  Product : Product
  Product1 : Product
  Sum : Sum  Inputs=|++
  Sum2 : Sum  Inputs=+-
  Filtered : Outport
  wires:
  w_cutoff/1 -> Divide/1
  dt/1 -> Divide/2
  Divide/1 -> Gain/1
  Raw/1 -> Product/1
  Product/1 -> Sum/1
  Sum/1 -> Delay/1, Filtered/1
  Product1/1 -> Sum/2
  Gain/1 -> Exp/1
  Exp/1 -> Product1/1, Sum2/2  "Alpha"
  Constant1/1 -> Sum2/1
  Sum2/1 -> Product/2
  Delay/1 -> Product1/2

== system ADCS_r2017b_may6/Flight Software/Subsystems/Sensor Processing/Discrete Low Pass Filter2 ==
  Raw : Inport
  w_cutoff : Inport  Port=2
  dt : Inport  Port=3
  Constant1 : Constant
  Delay : Delay  DelayLength=1  InitialCondition=0
  Divide : Product  Inputs=**
  Exp : Math  SaturateOnIntegerOverflow=on
  Gain : Gain  Gain=-1
  Product : Product
  Product1 : Product
  Sum : Sum  Inputs=|++
  Sum2 : Sum  Inputs=+-
  Filtered : Outport
  wires:
  w_cutoff/1 -> Divide/1
  dt/1 -> Divide/2
  Divide/1 -> Gain/1
  Raw/1 -> Product/1
  Product/1 -> Sum/1
  Sum/1 -> Delay/1, Filtered/1
  Product1/1 -> Sum/2
  Gain/1 -> Exp/1
  Exp/1 -> Product1/1, Sum2/2  "Alpha"
  Constant1/1 -> Sum2/1
  Sum2/1 -> Product/2
  Delay/1 -> Product1/2

== system ADCS_r2017b_may6/Flight Software/Subsystems/Sensor Processing/Discrete Low Pass Filter3 ==
  Raw : Inport
  w_cutoff : Inport  Port=2
  dt : Inport  Port=3
  Constant1 : Constant
  Delay : Delay  DelayLength=1  InitialCondition=0
  Divide : Product  Inputs=**
  Exp : Math  SaturateOnIntegerOverflow=on
  Gain : Gain  Gain=-1
  Product : Product
  Product1 : Product
  Sum : Sum  Inputs=|++
  Sum2 : Sum  Inputs=+-
  Filtered : Outport
  wires:
  w_cutoff/1 -> Divide/1
  dt/1 -> Divide/2
  Divide/1 -> Gain/1
  Raw/1 -> Product/1
  Product/1 -> Sum/1
  Sum/1 -> Delay/1, Filtered/1
  Product1/1 -> Sum/2
  Gain/1 -> Exp/1
  Exp/1 -> Product1/1, Sum2/2  "Alpha"
  Constant1/1 -> Sum2/1
  Sum2/1 -> Product/2
  Delay/1 -> Product1/2

== system ADCS_r2017b_may6/Satellite Simulator/External Forces and Torques/External Torques/Grav gradient earth ==
  r_eci : Inport
  R_eci2body : Inport  Port=2
  3x3 Cross Product : sharedutil/3x3 Cross Product  aMode=aMode
      settings: SourceProductBaseCode=AE
  Constant : Constant  Value=SC.mass_properties.inertia
  Constant1 : Constant  Value=SS.constants.GM_Earth
  MATLAB Function : MATLAB Function  TreatAsAtomicUnit=on
  Matrix Multiply : Product  Multiplication=Matrix(*)
  Matrix Multiply1 : Product  Multiplication=Matrix(*)
  Normalize Vector : vrlib/Utilities/Normalize Vector  maxzero=0
      settings: SourceProductName=Simulink 3D Animation  SourceProductBaseCode=VR
  Torque_body : Outport
  wires:
  R_eci2body/1 -> Matrix Multiply/1
  r_eci/1 -> MATLAB Function/2(r_eci), Matrix Multiply/2
  Matrix Multiply/1 -> Normalize Vector/1
  Constant/1 -> Matrix Multiply1/1
  Normalize Vector/1 -> 3x3 Cross Product/1, Matrix Multiply1/2
  Matrix Multiply1/1 -> 3x3 Cross Product/2
  3x3 Cross Product/1 -> MATLAB Function/1(rIr)
  Constant1/1 -> MATLAB Function/3(GM)
  MATLAB Function/1(tor) -> Torque_body/1

== system ADCS_r2017b_may6/Satellite Simulator/External Forces and Torques/External Torques/Grav gradient moon ==
  r_mci : Inport
  R_mci2body : Inport  Port=2
  3x3 Cross Product : sharedutil/3x3 Cross Product
      settings: SourceProductBaseCode=AE
  Constant : Constant  Value=SC.mass_properties.inertia
  Constant1 : Constant  Value=SS.constants.GM_Moon
  MATLAB Function : MATLAB Function  TreatAsAtomicUnit=on
  Matrix Multiply : Product  Multiplication=Matrix(*)
  Matrix Multiply1 : Product  Multiplication=Matrix(*)
  Normalize Vector : vrlib/Utilities/Normalize Vector  maxzero=0
      settings: SourceProductName=Simulink 3D Animation  SourceProductBaseCode=VR
  Torque_body : Outport
  wires:
  R_mci2body/1 -> Matrix Multiply/1
  r_mci/1 -> MATLAB Function/2(r_mci), Matrix Multiply/2
  Matrix Multiply/1 -> Normalize Vector/1
  Constant/1 -> Matrix Multiply1/1
  Normalize Vector/1 -> 3x3 Cross Product/1, Matrix Multiply1/2
  Matrix Multiply1/1 -> 3x3 Cross Product/2
  3x3 Cross Product/1 -> MATLAB Function/1(rIr)
  Constant1/1 -> MATLAB Function/3(GM)
  MATLAB Function/1(tor) -> Torque_body/1

== system ADCS_r2017b_may6/Satellite Simulator/Kinematics/Position Kinematics/Adams Bashforth Integration ==
  x_initial : Inport
  x_dot : Inport  Port=2
  dt : Inport  Port=3
  Delay : Delay  DelayLength=1  InitialConditionSource=Input port  InitialCondition=0
      settings: InputPortMap=u0,p4
  Delay1 : Delay  DelayLength=1  InitialConditionSource=Input port  InitialCondition=0
      settings: InputPortMap=u0,p4
  Delay2 : Delay  DelayLength=1  InitialConditionSource=Input port  InitialCondition=0
      settings: InputPortMap=u0,p4
  Gain : Gain  Gain=23/12
  Gain1 : Gain  Gain=-16/12
  Gain2 : Gain  Gain=5/12
  Product : Product
  Sum : Sum  Inputs=|++
  Sum1 : Sum  Inputs=+++
  x : Outport
  wires:
  x_initial/1 -> Delay/2
  Delay/1 -> Sum/1
  Sum/1 -> Delay/1, x/1
  Delay1/1 -> Delay2/1, Gain1/1
  x_dot/1 -> Delay2/2, Delay1/2, Delay1/1, Gain/1
  Gain1/1 -> Sum1/2
  Gain/1 -> Sum1/1
  Gain2/1 -> Sum1/3
  Sum1/1 -> Product/1
  dt/1 -> Product/2
  Product/1 -> Sum/2
  Delay2/1 -> Gain2/1

== system ADCS_r2017b_may6/Satellite Simulator/Kinematics/Position Kinematics/Adams Bashforth Integration1 ==
  x_initial : Inport
  x_dot : Inport  Port=2
  dt : Inport  Port=3
  Delay : Delay  DelayLength=1  InitialConditionSource=Input port  InitialCondition=0
      settings: InputPortMap=u0,p4
  Delay1 : Delay  DelayLength=1  InitialConditionSource=Input port  InitialCondition=0
      settings: InputPortMap=u0,p4
  Delay2 : Delay  DelayLength=1  InitialConditionSource=Input port  InitialCondition=0
      settings: InputPortMap=u0,p4
  Gain : Gain  Gain=23/12
  Gain1 : Gain  Gain=-16/12
  Gain2 : Gain  Gain=5/12
  Product : Product
  Sum : Sum  Inputs=|++
  Sum1 : Sum  Inputs=+++
  x : Outport
  wires:
  x_initial/1 -> Delay/2
  Delay/1 -> Sum/1
  Sum/1 -> Delay/1, x/1
  Delay1/1 -> Delay2/1, Gain1/1
  x_dot/1 -> Delay2/2, Delay1/2, Delay1/1, Gain/1
  Gain1/1 -> Sum1/2
  Gain/1 -> Sum1/1
  Gain2/1 -> Sum1/3
  Sum1/1 -> Product/1
  dt/1 -> Product/2
  Product/1 -> Sum/2
  Delay2/1 -> Gain2/1

== system ADCS_r2017b_may6/Satellite Simulator/Kinematics/Rotation Kinematics/Adams Bashforth Integration ==
  x_initial : Inport
  x_dot : Inport  Port=2
  dt : Inport  Port=3
  Delay : Delay  DelayLength=1  InitialConditionSource=Input port  InitialCondition=0
      settings: InputPortMap=u0,p4
  Delay1 : Delay  DelayLength=1  InitialConditionSource=Input port  InitialCondition=0
      settings: InputPortMap=u0,p4
  Delay2 : Delay  DelayLength=1  InitialConditionSource=Input port  InitialCondition=0
      settings: InputPortMap=u0,p4
  Gain : Gain  Gain=23/12
  Gain1 : Gain  Gain=-16/12
  Gain2 : Gain  Gain=5/12
  Product : Product
  Sum : Sum  Inputs=|++
  Sum1 : Sum  Inputs=+++
  x : Outport
  wires:
  x_initial/1 -> Delay/2
  Delay/1 -> Sum/1
  Sum/1 -> Delay/1, x/1
  Delay1/1 -> Delay2/1, Gain1/1
  x_dot/1 -> Delay2/2, Delay1/2, Delay1/1, Gain/1
  Gain1/1 -> Sum1/2
  Gain/1 -> Sum1/1
  Gain2/1 -> Sum1/3
  Sum1/1 -> Product/1
  dt/1 -> Product/2
  Product/1 -> Sum/2
  Delay2/1 -> Gain2/1

== system ADCS_r2017b_may6/Satellite Simulator/Kinematics/Rotation Kinematics/Adams Bashforth Integration1 ==
  x_initial : Inport
  x_dot : Inport  Port=2
  dt : Inport  Port=3
  Delay : Delay  DelayLength=1  InitialConditionSource=Input port  InitialCondition=0
      settings: InputPortMap=u0,p4
  Delay1 : Delay  DelayLength=1  InitialConditionSource=Input port  InitialCondition=0
      settings: InputPortMap=u0,p4
  Delay2 : Delay  DelayLength=1  InitialConditionSource=Input port  InitialCondition=0
      settings: InputPortMap=u0,p4
  Gain : Gain  Gain=23/12
  Gain1 : Gain  Gain=-16/12
  Gain2 : Gain  Gain=5/12
  Product : Product
  Sum : Sum  Inputs=|++
  Sum1 : Sum  Inputs=+++
  x : Outport
  wires:
  x_initial/1 -> Delay/2
  Delay/1 -> Sum/1
  Sum/1 -> Delay/1, x/1
  Delay1/1 -> Delay2/1, Gain1/1
  x_dot/1 -> Delay2/2, Delay1/2, Delay1/1, Gain/1
  Gain1/1 -> Sum1/2
  Gain/1 -> Sum1/1
  Gain2/1 -> Sum1/3
  Sum1/1 -> Product/1
  dt/1 -> Product/2
  Product/1 -> Sum/2
  Delay2/1 -> Gain2/1

== matlab function ADCS_r2017b_may6/Flight Software/Subsystems/Sensor Processing/Process Gyro ==
  data: raw input; gyro output; gain input; offset input; rot input
function gyro = process_gyro(raw, gain, offset, rot)

temp = rot * raw;
gyro = gain * (temp - offset);

== matlab function ADCS_r2017b_may6/Flight Software/Subsystems/Mode Selection/MATLAB Function ==
  data: gyro input; gains output; eclipse input; JD input; mode output; a input; b input; c input; d input; e input; f input
function [gains, mode]  = Mode_Logic(gyro, eclipse, JD, a,b,c,d,e,f)

gains = [1;1;1];
mode = 1;

%switch case, determine what part of mission we are in

== matlab function ADCS_r2017b_may6/Flight Software/Subsystems/Sensor Processing/Process Gyro1 ==
  data: raw input; sun_dir output; gain input; offset input; eclipse output; threshold input
function [sun_dir, eclipse] = process_sun(raw, gain, offset, threshold)
n = length(raw); %number of sun sensors
sun = zeros(n,1);
for i=1:length(raw)
    sun(i) = gain(i) * (raw(i) - offset(i));
end

%discuss advantages of different ways of turning sun measurements to direction
sun_x = sun(1)-sun(2);
sun_y = sun(3)-sun(4);
sun_z = sun(5)-sun(6);

sun_dir = [sun_x; sun_y; sun_z];
sun_dir = sun_dir/norm(sun_dir);

eclipse = 0;
if (sum(abs(sun < threshold)))
    eclipse = 1;
end

== matlab function ADCS_r2017b_may6/Satellite Simulator/External Forces and Torques/MATLAB Function ==
  data: I input; M output; GM input; rECI input; R_eci2principal input
function M = gravityGradient(I, GM, rECI, R_eci2principal)
% Expressed in principal axes. The c vector is the position vector of the
% satellite expressed in principal axes.

R = norm(rECI);
c = R_eci2principal*rECI;

Ix = I(1,1);
Iy = I(2,2);
Iz = I(3,3);
cx = c(1);
cy = c(2);
cz = c(3);

M = zeros(3,1);
M(1) = 3*GM/R^3 * (Iz - Iy)*cy*cz;
M(2) = 3*GM/R^3 * (Ix - Iz)*cz*cx;
M(3) = 3*GM/R^3 * (Iy - Ix)*cx*cy;
end

== matlab function ADCS_r2017b_may6/Satellite Simulator/External Forces and Torques/Gravity/Earth Gravity ==
  data: r_eci input; f_Earth output; GM_Earth input
function f_Earth = accelPointMass(r_eci, GM_Earth)
f_Earth = -GM_Earth*r_eci./norm(r_eci)^3;
end

== matlab function ADCS_r2017b_may6/Satellite Simulator/External Forces and Torques/Gravity/Moon Gravity ==
  data: r_mci input; f_Moon output; GM_Moon input
function f_Moon = accelPointMass(r_mci, GM_Moon)
f_Moon = -GM_Moon*r_mci./norm(r_mci)^3;
end

== matlab function ADCS_r2017b_may6/Satellite Simulator/Kinematics/Calc Coordinate Transforms/Calc_R_eci2body ==
  data: q input; R_eci2body output
function R_eci2body = fcn(q)
eta=q(4);
e1=q(1);
e2=q(2);
e3=q(3);

R_eci2body = [e1^2-e2^2-e3^2+eta^2, 2*(e1*e2+eta*e3),        2*(e1*e3-eta*e2);
              2*(e1*e2-eta*e3),     -1*e1^2+e2^2-e3^2+eta^2, 2*(e2*e3+eta*e1);
              2*(e1*e3+eta*e2),     2*(e2*e3-eta*e1),        -1*e1^2-e2^2+e3^2+eta^2];
          
end

== matlab function ADCS_r2017b_may6/Satellite Simulator/External Forces and Torques/Gravity/Sun Gravity ==
  data: r_hci input; f_Sun output; GM_Sun input
function f_Sun = accelPointMass(r_hci, GM_Sun)
f_Sun = -GM_Sun*r_hci./norm(r_hci)^3;
end

== matlab function ADCS_r2017b_may6/Satellite Simulator/Kinematics/Calc Coordinate Transforms/Calc_R_eci2ecef ==
  data: JD_i input; R_eci2ecef output
function R_eci2ecef = fcn(JD_i)
%Based on Seidlemann's "Explanatory Supplment to the Astronomical Almanac" page 50
%Given the JD, will return the rotation matrix to convert R_eci to R_ecef
JD = floor(JD_i);
seconds_per_day = 24*60*60;
SSN = seconds_per_day*(JD_i-JD);
seconds_per_half_day = seconds_per_day/2;
days_per_Julian_century = 36525;
JD_epoch = 2451545.00; %JD of noon on Jan 1, 2000

c1 = JD-JD_epoch+(SSN/seconds_per_day);
c2 = c1/days_per_Julian_century;

p1 = 24110.54841;
p2 = 8640184.812866;
p3 = 0.093104;
p4 = -6.2*10^-6;

c3 = (p1)+(p2*c2)+(p3*c2*c2)+(p4*c2*c2*c2)+(SSN)-(seconds_per_half_day);

c4 = c3*pi/seconds_per_half_day;

c5 = mod(c4, 2*pi);

a1 = cos(c5);
a2 = sin(c5);
a3 = -1*a2;
a4 = 0;
a5 = 1;
A = [a1;a3;a4;a2;a1;a4;a4;a4;a5];

R_eci2ecef = reshape(A, 3,3);
end

== matlab function ADCS_r2017b_may6/Satellite Simulator/Kinematics/Calc Coordinate Transforms/ecef2geod ==
  data: h output; r_ecef input; phi output; lambda output
function [h,phi,lambda] = ecef2geod(r_ecef)
%note - r_ecef should be in meters
a = 6378137;        %earth radius, meters
e = 0.081819190842; %earth eccentricity

% Reference: function ecef2geodetic in Matlab
x = r_ecef(1);
y = r_ecef(2);
z = r_ecef(3);

% Ellipsoid constants
e2 = e ^ 2;   % Square of first eccentricity
ep2 = e2 / (1 - e2);     % Square of second eccentricity
f = 1 - sqrt(1 - e2);    % Flattening
b = a * (1 - f);         % Semiminor axis
% Longitude
lambda = atan2(y,x); %[rad]
% Distance from Z-axis
rho = hypot(x,y);
% Bowring's formula for initial parametric (beta) and geodetic (phi) latitudes
beta = atan2(z, (1 - f) * rho);
phi = atan2(z   + b * ep2 * sin(beta).^3,...
            rho - a * e2  * cos(beta).^3); %[rad]
% Fixed-point iteration with Bowring's formula
% (typically converges within two or three iterations)
betaNew = atan2((1 - f)*sin(phi), cos(phi));
count = 0;
while any(beta ~= betaNew) && count < 5
    beta = betaNew;
    phi = atan2(z   + b * ep2 * sin(beta).^3,...
                rho - a * e2  * cos(beta).^3);
    betaNew = atan2((1 - f)*sin(phi), cos(phi));
    count = count + 1;
end
% Calculate ellipsoidal height from the final value for latitude
sinphi = sin(phi);
N = a ./ sqrt(1 - e2 * sinphi.^2);
h = rho .* cos(phi) + (z + e2 * N .* sinphi) .* sinphi - N;

phi=phi*180/pi; %[deg]
lambda=lambda*180/pi; %[deg]
end

== matlab function ADCS_r2017b_may6/Satellite Simulator/Kinematics/Rotation Kinematics/calc_q_dot ==
  data: q input; q_dot output; w input
function q_dot   = fcn(q, w)

wx = w(1); wy = w(2); wz = w(3);
OMEGA = [   0,    wz, -1*wy, wx;
        -1*wz,     0,    wx, wy;
           wy, -1*wx,     0, wz;
        -1*wx, -1*wy, -1*wz,  0];
q_dot = 0.5*OMEGA*q;
